simulink model "EMS_Stateflow_Example"  (R2025a)
settings: Solver=FixedStepDiscrete  StartTime=0.0  StopTime=0.01  FixedStep=0.01  RelTol=1e-3
undefined symbols (not defined in the file): Ibat_max, SOC_max, SOC_min
settings Model: Creator=Limingyu  LastModifiedBy=Limingyu

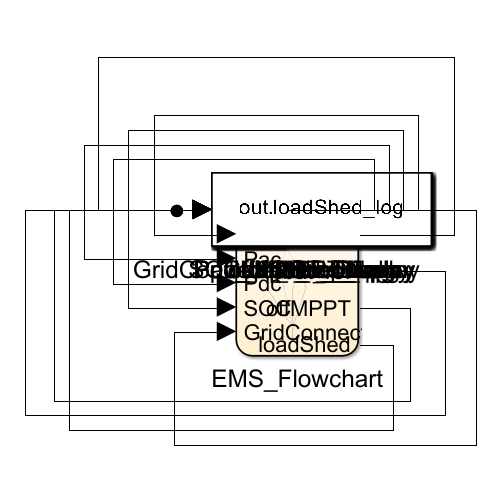
[thumbnail: Simulink's stored preview of the top-level diagram]
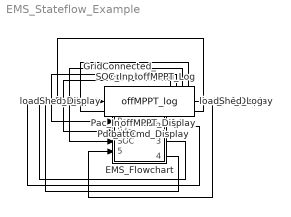
== system EMS_Stateflow_Example ==
  EMS_Flowchart : Stateflow chart  TreatAsAtomicUnit=on
  GridConnected_Input : Constant  Value=false  OutDataTypeStr=boolean
  Ibat_ref_Display : Display
  Ibat_ref_Log : ToWorkspace  VariableName=Ibat_ref_log  SaveFormat=Timeseries
  Pac_Input : Constant  Value=100e3
  Pdc_Input : Constant  Value=0
  Ppv_Input : Constant  Value=0
  SOC_Input : Constant  Value=50
  battCmd_Display : Display
  battCmd_Log : ToWorkspace  VariableName=battCmd_log  SaveFormat=Timeseries
  loadShed_Display : Display
  loadShed_Log : ToWorkspace  VariableName=loadShed_log  SaveFormat=Timeseries
  offMPPT_Display : Display
  offMPPT_Log : ToWorkspace  VariableName=offMPPT_log  SaveFormat=Timeseries
  wires:
  Ppv_Input/1 -> EMS_Flowchart/1(Ppv)
  Pac_Input/1 -> EMS_Flowchart/2(Pac)
  Pdc_Input/1 -> EMS_Flowchart/3(Pdc)
  SOC_Input/1 -> EMS_Flowchart/4(SOC)
  GridConnected_Input/1 -> EMS_Flowchart/5(GridConnected)
  EMS_Flowchart/1(battCmd) -> battCmd_Log/1, battCmd_Display/1
  EMS_Flowchart/2(Ibat_ref) -> Ibat_ref_Log/1, Ibat_ref_Display/1
  EMS_Flowchart/3(offMPPT) -> offMPPT_Log/1, offMPPT_Display/1
  EMS_Flowchart/4(loadShed) -> loadShed_Log/1, loadShed_Display/1

== stateflow chart EMS_Stateflow_Example/EMS_Flowchart ==
  (default) -> (junction 16) : {battCmd = 0.0;
      | Ibat_ref = 0.0;
      | offMPPT = false;
      | loadShed = false;
      | Pnet = Ppv - Pac - Pdc;
      | SOC_mid = 0.5 * (SOC_min + SOC_max);
      | frac = (SOC - SOC_min) / (SOC_max - SOC_min);
      | frac = min(max(frac,0.0),1.0);}
  (junction 16) -> (junction 19) [order 2]
  (junction 16) -> (junction 17) [order 1] : [GridConnected == true]
  (junction 17) -> (junction 18) [order 2]
  (junction 19) -> (junction 20) [order 1] : [Pnet < 0.0]
  (junction 19) -> (junction 21) [order 2]
  (junction 17) -> (junction 22) [order 1] : [SOC < SOC_mid]{battCmd = -1.0;}
  (junction 18) -> (junction 22) [order 1] : [Pnet < 0.0 && SOC > SOC_min]{battCmd = 1.0;}
  (junction 18) -> (junction 22) [order 2] : {battCmd = 0.0;}
  (junction 21) -> (junction 22) [order 1] : [SOC < SOC_max]{battCmd = -1.0;}
  (junction 21) -> (junction 22) [order 2] : {battCmd = 0.0;
      | offMPPT = true;}
  (junction 20) -> (junction 22) [order 1] : [SOC > SOC_min]{battCmd = 1.0;}
  (junction 20) -> (junction 22) [order 2] : {battCmd = 0.0;
      | loadShed = true;}
  (junction 22) -> (junction 23) [order 1] : [battCmd == 1.0]{Ibat_ref = Ibat_max * frac;}
  (junction 22) -> (junction 23) [order 2] : [battCmd == -1.0]{Ibat_ref = -Ibat_max * (1.0 - frac);}
  (junction 22) -> (junction 23) [order 3] : {Ibat_ref = 0.0;}
  data: Ppv input double; Pac input double; Pdc input double; SOC input double; GridConnected input boolean; battCmd output double; Ibat_ref output double; offMPPT output boolean; loadShed output boolean; SOC_min parameter double; SOC_max parameter double; Ibat_max parameter double; Pnet local double; SOC_mid local double; frac local double
